simulink model "DifferetialDrive_MotorControl_Traj"  (R2024b)
settings: Solver=VariableStepAuto  StartTime=0.0  StopTime=50  RelTol=1e-3
values from neighbouring files (symbols this model uses):
  ki1_vel = 0.35    [DifferentialDrive_MotorControl.m]
  ki2_vel = 0.35    [DifferentialDrive_MotorControl.m]
  kp1_vel = 0.12    [DifferentialDrive_MotorControl.m]
  kp2_vel = 0.12    [DifferentialDrive_MotorControl.m]
  Kp_L = 1    [DifferentialDrive_MotorControl.m]
  Kp_theta = 1    [DifferentialDrive_MotorControl.m]
  ku1 = 10    [DifferentialDrive_MotorControl.m]
  ku2 = 10    [DifferentialDrive_MotorControl.m]
  MM = [1/2 1/2; -1/dd 1/dd].*rr    [DifferentialDrive_MotorControl.m]
  MMinv = [1 -dd/2; 1  dd/2]./rr    [DifferentialDrive_MotorControl.m]
  MoveTime = 5    [DifferentialDrive_MotorControl.m]
  o_sat = 2    [DifferentialDrive_MotorControl.m]
  tau1 = 0.14    [DifferentialDrive_MotorControl.m]
  tau2 = 0.14    [DifferentialDrive_MotorControl.m]
  Ts = 0.1    [DifferentialDrive_MotorControl.m]
  Ts_vel = 1/200    (= 0.005)    [DifferentialDrive_MotorControl.m]
  v_sat = 8    [DifferentialDrive_MotorControl.m]
libraries: slpidlib x2, robotmobilelib x1, simulink x1
settings Model: Creator=ttsao  LastModifiedBy=ssw71

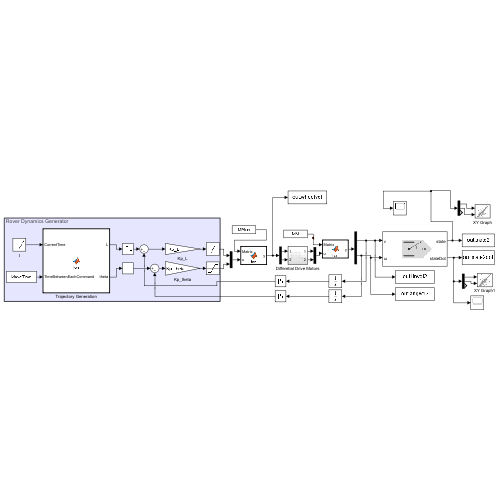
[thumbnail: Simulink's stored preview of the top-level diagram]
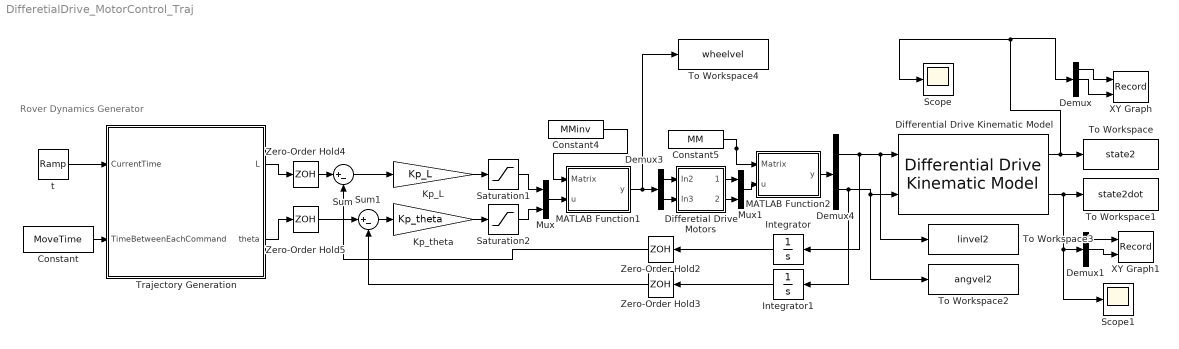
== system DifferetialDrive_MotorControl_Traj ==
  note: Rover Dynamics Generator
  Constant : Constant  Value=MoveTime
  Constant4 : Constant  Value=MMinv
  Constant5 : Constant  Value=MM
  Demux : Demux  Outputs=3
  Demux1 : Demux  Outputs=3
  Demux3 : Demux  Outputs=2
  Demux4 : Demux  Outputs=2
  Differential Drive Kinematic Model : robotmobilelib/Differential Drive Kinematic Model  VehicleInputs=Vehicle Speed & Heading Angular Velocity  WheelRadius=rr  WheelSpeedRange=[-inf inf]  TrackWidth=dd  InitialState=[0; 0; 0]  SimulateUsing=Interpreted execution
  Differetial Drive Motors : Subsystem
  Integrator : Integrator
  Integrator1 : Integrator
  Kp_L : Gain  Gain=Kp_L
  Kp_theta : Gain  Gain=Kp_theta
  MATLAB Function1 : MATLAB Function  TreatAsAtomicUnit=on
  MATLAB Function2 : MATLAB Function  TreatAsAtomicUnit=on
  Mux : Mux  Inputs=2
  Mux1 : Mux  Inputs=2
  Saturation1 : Saturate  UpperLimit=v_sat  LowerLimit=-v_sat
  Saturation2 : Saturate  UpperLimit=o_sat  LowerLimit=-o_sat
  Scope : Scope
  Scope1 : Scope
  Sum : Sum  Inputs=|+-
  Sum1 : Sum  Inputs=|+-
  To Workspace : ToWorkspace  VariableName=state2  SaveFormat=Timeseries  SampleTime=-1
  To Workspace1 : ToWorkspace  VariableName=state2dot  SaveFormat=Timeseries  SampleTime=-1
  To Workspace2 : ToWorkspace  VariableName=angvel2  SaveFormat=Timeseries  SampleTime=-1
  To Workspace3 : ToWorkspace  VariableName=linvel2  SaveFormat=Timeseries  SampleTime=-1
  To Workspace4 : ToWorkspace  VariableName=wheelvel  SaveFormat=Timeseries  SampleTime=-1
  Trajectory Generation : MATLAB Function  TreatAsAtomicUnit=on
  XY Graph : Record  FileSettingsInternal="{\"entries\":[{\"content\":{\"excelSettings\":{\"content\":{},\"type\":\"Streamout.ExcelSettings\"}},\"type\":\"Streamout.FileSettingStorage\",\"uuid\":\"\"}],\"packageUris\":[\"http:\\/\\/schema.mathworks.com\\/mf0\\/streamout_blocks\\/R2020a\"],\"version\":\"1.0\"}"  Layout=[1 1]  SignalsInternal="{\"entries\":[{\"content\":{\"signals\":[{\"content\":{\"blockPath\":[],\"dimensions\":[1],\"domain\":\"\",\"lineColor\":\"#22b573\",\"lineWidth\":2,\"plots\":[ 1 ],\"port\":1,\"sid\":[\"\"],\"signalID\":1,\"signalName\":\"Demux:1\"},\"type\":\"RecordBlkView.Signal\",\"uuid\":\"\"},{\"content\":{\"blockPath\":[],\"dimensions\":[1],\"domain\":\"\",\"lineColor\":\"#0072bd\",\"lineWidth\":2,\"plots\":[ 1 ],\"port\":2,\"sid\":[\"\"],\"signalID\":2,\"signalName\":\"Demux:2\"},\"type\":\"RecordBlkView.Signal\",\"uuid\":\"\"}]},\"type\":\"RecordBlkView.InputSignals\",\"uuid\":\"\"}],\"packageUris\":[\"http:\\/\\/schema.mathworks.com\\/mf0\\/streamout_blocks\\/R2020a\"],\"version\":\"1.0\"}"  VisualizationBindings="{\"xyplotplugin\":{\"info\":[{\"series\":[{\"bindingParametersList\":[{\"parameter\":\"X-Axis\",\"signalID\":1,\"signalName\":\"Demux:1\"},{\"parameter\":\"Y-Axis\",\"signalID\":2,\"signalName\":\"Demux:2\"}],\"seriesID\":0}],\"subplotID\":1}]}}"  CompatibilityTag=XY
  XY Graph1 : Record  Filename=recording_velpcity.mldatx  FileSettingsInternal="{\"entries\":[{\"content\":{\"excelSettings\":{\"content\":{},\"type\":\"Streamout.ExcelSettings\"}},\"type\":\"Streamout.FileSettingStorage\",\"uuid\":\"\"}],\"packageUris\":[\"http:\\/\\/schema.mathworks.com\\/mf0\\/streamout_blocks\\/R2020a\"],\"version\":\"1.0\"}"  Layout=[1 1]  SignalsInternal="{\"entries\":[{\"content\":{\"signals\":[{\"content\":{\"blockPath\":[],\"dimensions\":[1],\"domain\":\"\",\"lineColor\":\"#a2142f\",\"plots\":[ 1 ],\"port\":1,\"sid\":[\"\"],\"signalID\":1,\"signalName\":\"Demux1:1\"},\"type\":\"RecordBlkView.Signal\",\"uuid\":\"\"},{\"content\":{\"blockPath\":[],\"dimensions\":[1],\"domain\":\"\",\"lineColor\":\"#139fff\",\"plots\":[ 1 ],\"port\":2,\"sid\":[\"\"],\"signalID\":2,\"signalName\":\"Demux1:2\"},\"type\":\"RecordBlkView.Signal\",\"uuid\":\"\"}]},\"type\":\"RecordBlkView.InputSignals\",\"uuid\":\"\"}],\"packageUris\":[\"http:\\/\\/schema.mathworks.com\\/mf0\\/streamout_blocks\\/R2020a\"],\"version\":\"1.0\"}"  VisualizationBindings="{\"xyplotplugin\":{\"info\":[{\"series\":[{\"bindingParametersList\":[{\"parameter\":\"X-Axis\",\"signalID\":1,\"signalName\":\"Demux1:1\"},{\"parameter\":\"Y-Axis\",\"signalID\":2,\"signalName\":\"Demux1:2\"}],\"seriesID\":0}],\"subplotID\":1}]}}"  CompatibilityTag=XY
  Zero-Order Hold{2..5} (4 alike) : ZeroOrderHold  SampleTime=Ts
  t : simulink/Sources/Ramp  slope=1  start=0  InitialOutput=0
  wires:
  Demux/1 -> XY Graph/1
  Demux/2 -> XY Graph/2
  Differential Drive Kinematic Model/1 -> To Workspace/1, Demux/1, Scope/1
  Demux3/1 -> Differetial Drive Motors/1(In2)
  Demux3/2 -> Differetial Drive Motors/2(In3)
  MATLAB Function1/1(y) -> Demux3/1, To Workspace4/1
  Mux/1 -> MATLAB Function1/2(u)
  Demux4/1 -> Differential Drive Kinematic Model/1, To Workspace3/1, Integrator/1
  MATLAB Function2/1(y) -> Demux4/1
  Differetial Drive Motors/1(Out2) -> Mux1/1
  Differetial Drive Motors/2(Out3) -> Mux1/2
  Constant4/1 -> MATLAB Function1/1(Matrix)
  Constant5/1 -> MATLAB Function2/1(Matrix)
  Mux1/1 -> MATLAB Function2/2(u)
  Demux4/2 -> To Workspace2/1, Differential Drive Kinematic Model/2, Integrator1/1
  Sum/1 -> Kp_L/1
  Integrator/1 -> Zero-Order Hold2/1
  Trajectory Generation/2(theta) -> Zero-Order Hold5/1
  Integrator1/1 -> Zero-Order Hold3/1
  Sum1/1 -> Kp_theta/1
  Zero-Order Hold2/1 -> Sum/2
  Zero-Order Hold3/1 -> Sum1/2
  Zero-Order Hold4/1 -> Sum/1
  Zero-Order Hold5/1 -> Sum1/1
  t/1 -> Trajectory Generation/1(CurrentTime)
  Constant/1 -> Trajectory Generation/2(TimeBetweenEachCommand)
  Demux1/1 -> XY Graph1/1
  Differential Drive Kinematic Model/2 -> To Workspace1/1, Scope1/1, Demux1/1
  Demux1/2 -> XY Graph1/2
  Trajectory Generation/1(L) -> Zero-Order Hold4/1
  Kp_L/1 -> Saturation1/1
  Saturation1/1 -> Mux/1
  Kp_theta/1 -> Saturation2/1
  Saturation2/1 -> Mux/2

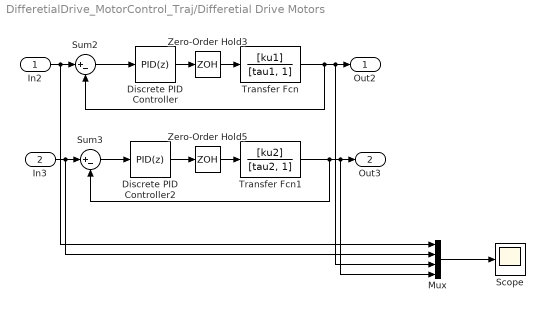
== system DifferetialDrive_MotorControl_Traj/Differetial Drive Motors ==
  In2 : Inport
  In3 : Inport  Port=2
  Discrete PID Controller : slpidlib/PID Controller  Controller=PID  Form=Parallel  TimeDomain=Discrete-time  UseExternalTs=off  SampleTime=Ts_vel  IntegratorMethod=Forward Euler  FilterMethod=Forward Euler  ControllerParametersSource=internal  P=kp1_vel  I=ki1_vel  UseKiTs=off  D=0  UseExternalDerivativeSource=off  N=100  UseFilter=on  TunerSelectOption=Transfer Function Based (PID Tuner App)  InitialConditionSource=internal  InitialConditionForIntegrator=0  InitialConditionForFilter=0  DifferentiatorICPrevScaledInput=0  ExternalReset=none  TrackingMode=off  Kt=1  LimitOutput=off  SatLimitsSource=internal  UpperSaturationLimit=inf  LowerSaturationLimit=-inf  LinearizeAsGain=off  AntiWindupMode=none  Kb=1  LimitIntegrator=off  UpperIntegratorSaturationLimit=inf  LowerIntegratorSaturationLimit=-inf  POutMin=[]  POutMax=[]  IOutMin=[]  IOutMax=[]  DOutMin=[]  DOutMax=[]  NOutMin=[]  NOutMax=[]  SumOutMin=[]  SumOutMax=[]  SaturationOutMin=[]  SaturationOutMax=[]  PParamMin=[]  PParamMax=[]  IParamMin=[]  IParamMax=[]  DParamMin=[]  DParamMax=[]  NParamMin=[]  NParamMax=[]  KbParamMin=[]  KbParamMax=[]  KtParamMin=[]  KtParamMax=[]  KbOutMin=[]  KbOutMax=[]  KtOutMin=[]  KtOutMax=[]  IntegratorOutMin=[]  IntegratorOutMax=[]  FilterOutMin=[]  FilterOutMax=[]  SumI1OutMin=[]  SumI1OutMax=[]  SumI2OutMin=[]  SumI2OutMax=[]  SumI3OutMin=[]  SumI3OutMax=[]  SumI4OutMin=[]  SumI4OutMax=[]  SumDOutMin=[]  SumDOutMax=[]  DifferentiatorOutMin=[]  DifferentiatorOutMax=[]  FilterDiffOutCoefMin=[]  FilterDiffOutCoefMax=[]  ReciprocalOutMin=[]  ReciprocalOutMax=[]  SumDenOutMin=[]  SumDenOutMax=[]  SumNumOutMin=[]  SumNumOutMax=[]  DivideOutMin=[]  DivideOutMax=[]  UdiffTsProdOutMin=[]  UdiffTsProdOutMax=[]  NTsProdOutMin=[]  NTsProdOutMax=[]  UintegralTsProdOutMin=[]  UintegralTsProdOutMax=[]  UngainTsProdOutMin=[]  UngainTsProdOutMax=[]  ClampingZeroOutDataTypeStr=Inherit: Inherit via back propagation  ClampingZeroOutMin=[]  ClampingZeroOutMax=[]  FilterDenConstantOutDataTypeStr=Inherit: Inherit via back propagation  FilterDenConstantOutMin=[]  FilterDenConstantOutMax=[]  PCopyOutDataTypeStr=Inherit: Inherit via back propagation  PCopyOutMin=[]  PCopyOutMax=[]  NCopyOutDataTypeStr=Inherit: Inherit via back propagation  NCopyOutMin=[]  NCopyOutMax=[]  IntegratorContinuousStateAttributes=''  IntegratorStateMustResolveToSignalObject=off  IntegratorRTWStateStorageClass=Auto  FilterContinuousStateAttributes=''  FilterStateMustResolveToSignalObject=off  FilterRTWStateStorageClass=Auto  ParallelPVariant=InternalParameters  IdealPVariant=Disabled  IVariant=InternalParameters  DVariant=InternalParameters  IntegratorVariant=Discrete  SatVariant=Disabled  AWVariant=Passthrough  PCopyVariant=Disabled  TRVariant=Disabled  FdbkBlocksVariant=Forward  IdealPFdbkVariant=Disabled  SatFdbkVariant=Disabled  DerivativeFilterVariant=ForwardEulerFilter  NVariant=InternalParameters  NCopyVariant=Disabled  FilterICVariant=InternalICsFilter  IntegratorICVariant=InternalICs  ExternalResetVariant=Disabled  TRSumVariant=Passthrough  SumFdbkVariant=Disabled  SumVariant=Sum_PID  TsampFilterVariant=InternalTs  TsampNgainVariant=Passthrough  TsampIntegralVariant=Disabled_SignalSpec  ExternalSaturationOutDataTypeStr=Inherit: Same as second input  DerivativeSourceVariant=ErrorSignal  PreIntVariant=InternalPreInt
      settings: LibrarySourceBlock=simulink/Discrete/Discrete PID Controller
  Discrete PID Controller2 : slpidlib/PID Controller  Controller=PID  Form=Parallel  TimeDomain=Discrete-time  UseExternalTs=off  SampleTime=Ts_vel  IntegratorMethod=Forward Euler  FilterMethod=Forward Euler  ControllerParametersSource=internal  P=kp2_vel  I=ki2_vel  UseKiTs=off  D=0  UseExternalDerivativeSource=off  N=100  UseFilter=on  TunerSelectOption=Transfer Function Based (PID Tuner App)  InitialConditionSource=internal  InitialConditionForIntegrator=0  InitialConditionForFilter=0  DifferentiatorICPrevScaledInput=0  ExternalReset=none  TrackingMode=off  Kt=1  LimitOutput=off  SatLimitsSource=internal  UpperSaturationLimit=inf  LowerSaturationLimit=-inf  LinearizeAsGain=off  AntiWindupMode=none  Kb=1  LimitIntegrator=off  UpperIntegratorSaturationLimit=inf  LowerIntegratorSaturationLimit=-inf  POutMin=[]  POutMax=[]  IOutMin=[]  IOutMax=[]  DOutMin=[]  DOutMax=[]  NOutMin=[]  NOutMax=[]  SumOutMin=[]  SumOutMax=[]  SaturationOutMin=[]  SaturationOutMax=[]  PParamMin=[]  PParamMax=[]  IParamMin=[]  IParamMax=[]  DParamMin=[]  DParamMax=[]  NParamMin=[]  NParamMax=[]  KbParamMin=[]  KbParamMax=[]  KtParamMin=[]  KtParamMax=[]  KbOutMin=[]  KbOutMax=[]  KtOutMin=[]  KtOutMax=[]  IntegratorOutMin=[]  IntegratorOutMax=[]  FilterOutMin=[]  FilterOutMax=[]  SumI1OutMin=[]  SumI1OutMax=[]  SumI2OutMin=[]  SumI2OutMax=[]  SumI3OutMin=[]  SumI3OutMax=[]  SumI4OutMin=[]  SumI4OutMax=[]  SumDOutMin=[]  SumDOutMax=[]  DifferentiatorOutMin=[]  DifferentiatorOutMax=[]  FilterDiffOutCoefMin=[]  FilterDiffOutCoefMax=[]  ReciprocalOutMin=[]  ReciprocalOutMax=[]  SumDenOutMin=[]  SumDenOutMax=[]  SumNumOutMin=[]  SumNumOutMax=[]  DivideOutMin=[]  DivideOutMax=[]  UdiffTsProdOutMin=[]  UdiffTsProdOutMax=[]  NTsProdOutMin=[]  NTsProdOutMax=[]  UintegralTsProdOutMin=[]  UintegralTsProdOutMax=[]  UngainTsProdOutMin=[]  UngainTsProdOutMax=[]  ClampingZeroOutDataTypeStr=Inherit: Inherit via back propagation  ClampingZeroOutMin=[]  ClampingZeroOutMax=[]  FilterDenConstantOutDataTypeStr=Inherit: Inherit via back propagation  FilterDenConstantOutMin=[]  FilterDenConstantOutMax=[]  PCopyOutDataTypeStr=Inherit: Inherit via back propagation  PCopyOutMin=[]  PCopyOutMax=[]  NCopyOutDataTypeStr=Inherit: Inherit via back propagation  NCopyOutMin=[]  NCopyOutMax=[]  IntegratorContinuousStateAttributes=''  IntegratorStateMustResolveToSignalObject=off  IntegratorRTWStateStorageClass=Auto  FilterContinuousStateAttributes=''  FilterStateMustResolveToSignalObject=off  FilterRTWStateStorageClass=Auto  ParallelPVariant=InternalParameters  IdealPVariant=Disabled  IVariant=InternalParameters  DVariant=InternalParameters  IntegratorVariant=Discrete  SatVariant=Disabled  AWVariant=Passthrough  PCopyVariant=Disabled  TRVariant=Disabled  FdbkBlocksVariant=Forward  IdealPFdbkVariant=Disabled  SatFdbkVariant=Disabled  DerivativeFilterVariant=ForwardEulerFilter  NVariant=InternalParameters  NCopyVariant=Disabled  FilterICVariant=InternalICsFilter  IntegratorICVariant=InternalICs  ExternalResetVariant=Disabled  TRSumVariant=Passthrough  SumFdbkVariant=Disabled  SumVariant=Sum_PID  TsampFilterVariant=InternalTs  TsampNgainVariant=Passthrough  TsampIntegralVariant=Disabled_SignalSpec  ExternalSaturationOutDataTypeStr=Inherit: Same as second input  DerivativeSourceVariant=ErrorSignal  PreIntVariant=InternalPreInt
      settings: LibrarySourceBlock=simulink/Discrete/Discrete PID Controller
  Mux : Mux
  Scope : Scope
  Sum2 : Sum  Inputs=|+-
  Sum3 : Sum  Inputs=|+-
  Transfer Fcn : TransferFcn  Numerator=[ku1]  Denominator=[tau1, 1]
  Transfer Fcn1 : TransferFcn  Numerator=[ku2]  Denominator=[tau2, 1]
  Zero-Order Hold3 : ZeroOrderHold  SampleTime=-1
  Zero-Order Hold5 : ZeroOrderHold  SampleTime=-1
  Out2 : Outport
  Out3 : Outport  Port=2
  wires:
  Sum3/1 -> Discrete PID Controller2/1
  Discrete PID Controller2/1 -> Zero-Order Hold5/1
  In3/1 -> Mux/2, Sum3/1
  Zero-Order Hold5/1 -> Transfer Fcn1/1
  Sum2/1 -> Discrete PID Controller/1
  Zero-Order Hold3/1 -> Transfer Fcn/1
  Discrete PID Controller/1 -> Zero-Order Hold3/1
  Transfer Fcn/1 -> Sum2/2, Mux/3, Out2/1
  In2/1 -> Mux/1, Sum2/1
  Mux/1 -> Scope/1
  Transfer Fcn1/1 -> Sum3/2, Mux/4, Out3/1

== matlab function DifferetialDrive_MotorControl_Traj/MATLAB Function1 ==
  data: Matrix input; u input; y output
function y = fcn(Matrix,u)

y = Matrix* u;

== matlab function DifferetialDrive_MotorControl_Traj/Trajectory Generation ==
  data: L output; theta output; CurrentTime input; TimeBetweenEachCommand input
function [L, theta]= fcn(CurrentTime, TimeBetweenEachCommand)

L_array     = [0 10 20   20   40]; % Finish this distance commands array
Theta_array = [0  0  0 pi/2 pi/2]; % Finish this angle commands array


index = floor(CurrentTime/TimeBetweenEachCommand) + 1;
if index>length(L_array)
    index = length(L_array);
end
L = L_array(index);
theta = Theta_array(index);

== matlab function DifferetialDrive_MotorControl_Traj/MATLAB Function2 ==
  data: Matrix input; u input; y output
function y = fcn(Matrix,u)

y = Matrix* u;
